simulink subsystem "Leds_Colision"  (R2024b)
settings: Solver=VariableStepAuto  StartTime=0.0  StopTime=10.0  RelTol=1e-3
settings Model: Creator=Chenfu  LastModifiedBy=Chenfu

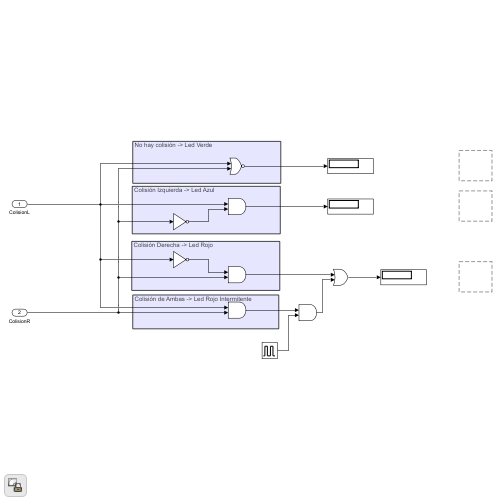
[thumbnail: Simulink's stored preview of the top-level diagram]
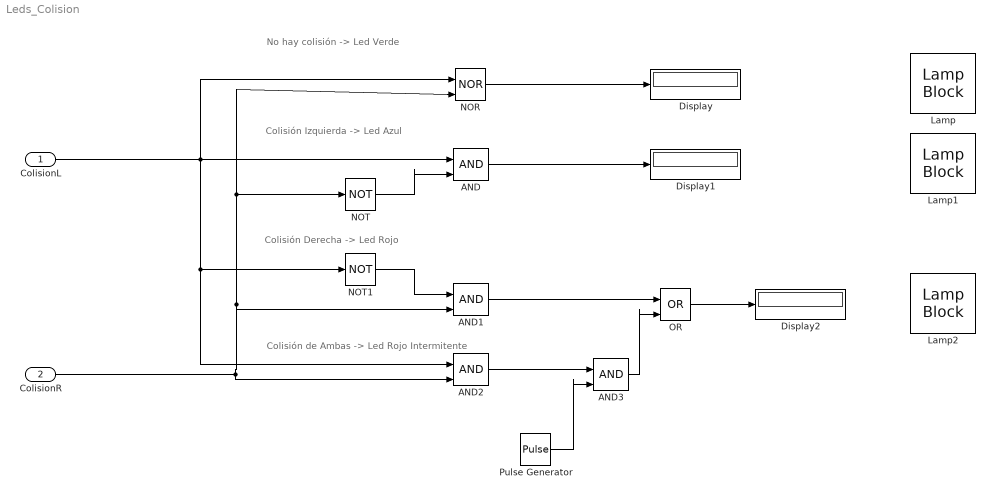
== system Leds_Colision ==
  note: Colisión de Ambas -> Led Rojo Intermitente
  note: Colisión Derecha -> Led Rojo
  note: Colisión Izquierda -> Led Azul
  note: No hay colisión -> Led Verde
  ColisionL : Inport
  ColisionR : Inport  Port=2
  AND{,1..3} (4 alike) : Logic  IconShape=distinctive  AllPortsSameDT=off  OutDataTypeStr=boolean
  Display : Display
  Display1 : Display
  Display2 : Display
  Lamp : LampBlock  LabelPosition=Hide
  Lamp1 : LampBlock  LabelPosition=Hide
  Lamp2 : LampBlock  LabelPosition=Hide
  NOR : Logic  Operator=NOR  IconShape=distinctive  AllPortsSameDT=off  OutDataTypeStr=boolean
  NOT : Logic  Operator=NOT  IconShape=distinctive  AllPortsSameDT=off  OutDataTypeStr=boolean
  NOT1 : Logic  Operator=NOT  IconShape=distinctive  AllPortsSameDT=off  OutDataTypeStr=boolean
  OR : Logic  Operator=OR  IconShape=distinctive  AllPortsSameDT=off  OutDataTypeStr=boolean
  Pulse Generator : DiscretePulseGenerator  PulseType=Time based  Period=10  PulseWidth=5
  wires:
  ColisionL/1 -> NOT1/1, AND2/1, AND/1, NOR/1
  ColisionR/1 -> AND1/2, NOT/1, NOR/2, AND2/2
  NOT/1 -> AND/2
  NOT1/1 -> AND1/1
  AND2/1 -> AND3/1
  Pulse Generator/1 -> AND3/2
  AND1/1 -> OR/1
  AND3/1 -> OR/2
  OR/1 -> Display2/1
  AND/1 -> Display1/1
  NOR/1 -> Display/1
